simulink model "challenge1_2"  (R2022b)
settings: Solver=ode45  StartTime=0.0  StopTime=10  RelTol=1e-3
undefined symbols (not defined in the file or in its folder): awu, degs2rpm, der, end_step, pid, rpm2degs, sens, simul, Ts
libraries: simulink x4
settings Model: Creator=emanuelevitetta  LastModifiedBy=david

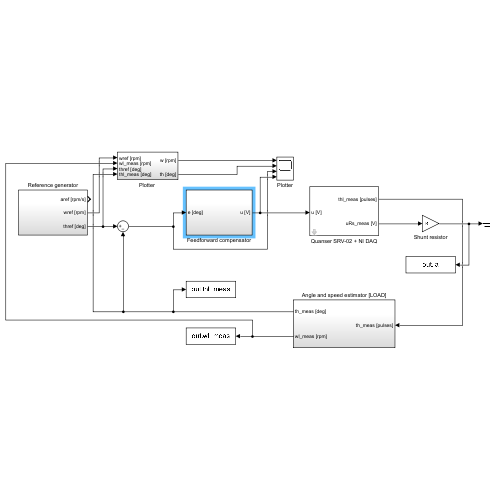
[thumbnail: Simulink's stored preview of the top-level diagram]
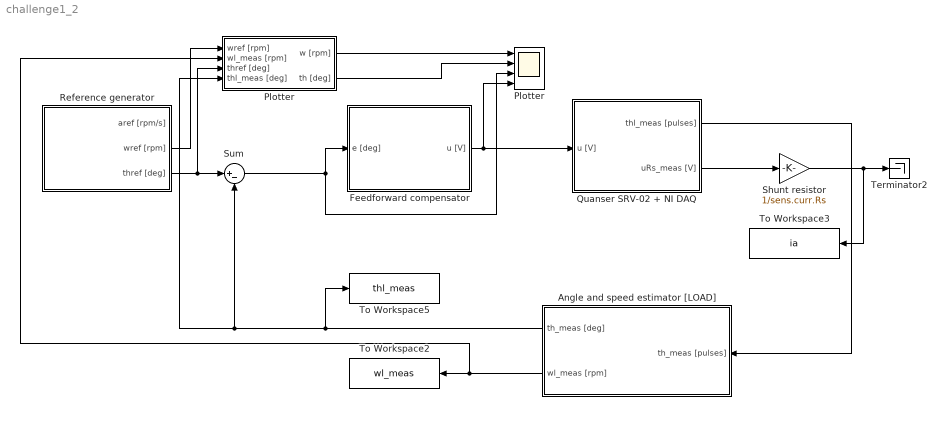
== system challenge1_2 ==
  Angle and speed estimator [LOAD] : Subsystem
  Feedforward compensator : Subsystem
  Plotter : Scope  NumInputPorts=4
  "Plotter " : Subsystem
  Quanser SRV-02 + NI DAQ : Subsystem  mask(Quanser SRV-02 (with inertial load) + NI DAQ){Ts=0.001, fricType=Coulomb + viscous}
      mask prompts: Ts "NI DAQ Sample Time:"; fricType "Friction model"
      mask help: Quanser SRV-02 (with inertial load) + NI DAQ model.
      mask init:
      | %%  Sensors data
      | 
      | %   shunt resistor
      | sens.curr.Rs = 0.5;                         %   resistance [Ohm]   
      | sens.curr.uRs_std = 0.01;                   %   voltage noise standard dev [V]                           
      | sens.curr.uRs_var = sens.curr.uRs_std^2;	%   voltage noise variance [V^2]
      | 
      | %   Hewlett-Packard HEDS-5540#A06 optical encoder
      | sens.enc.ppr = 500*4;                       %   pulses per rotation
      | sens.enc.pulse2deg = 360/sens.enc.ppr;      %   [pulses] -> [deg]
      | sens.enc.pulse2rad = 2*pi/sens.enc.ppr;     %   [pulses] -> [rad]
      | sens.enc.deg2pulse = sens.enc.ppr/360;      %   [deg] -> [pulses]
      | sens.enc.rad2pulse = sens.enc.ppr/2/pi;     %   [rad] -> [pulses]
      | 
      | 
      | %%  Data acquisition board (daq) data
      | 
      | %   NI PCI-6221 DAC data
      | daq.dac.bits = 16;                                  %   resolution (bits)
      | daq.dac.fs   = 10;                                  %   full scale 
      | daq.dac.q    = 2*daq.dac.fs/(2^daq.dac.bits-1);     %	quantization
      | 
      | %   NI PCI-6221 ADC data
      | daq.adc.bits = 16;                                  %   resolution (bits)
      | daq.adc.fs   = 10;                                  %   full scale (as set in SLDRT Analog Input block)
      | daq.adc.q    = 2*daq.adc.fs/(2^daq.adc.bits-1);     %   quantization
      mask Help:
      | Riccardo Antonello (antonello@dei.unipd.it)
      | 
      | April 24, 2020
      | 
      | Dept. of Information Engineering, University of Padova
      mask TypeOptions fricType: Coulomb + viscous | Karnopp
  Reference generator : Subsystem
  Shunt resistor : Gain  Gain=1/sens.curr.Rs
  Sum : Sum  Inputs=|+-
  Terminator2 : Terminator
  To Workspace2 : ToWorkspace  VariableName=wl_meas  SaveFormat=Structure With Time  SampleTime=Ts
  To Workspace3 : ToWorkspace  VariableName=ia  SaveFormat=Structure With Time  SampleTime=Ts
  To Workspace5 : ToWorkspace  VariableName=thl_meas  SaveFormat=Structure With Time  SampleTime=Ts
  wires:
  Quanser SRV-02 + NI DAQ/2(uRs_meas [V]) -> Shunt resistor/1
  Shunt resistor/1 -> To Workspace3/1, Terminator2/1
  Reference generator/3(thref [deg]) -> "Plotter "/3(thref [deg]), Sum/1
  Quanser SRV-02 + NI DAQ/1(thl_meas [pulses]) -> Angle and speed estimator [LOAD]/1(th_meas [pulses])
  Angle and speed estimator [LOAD]/1(th_meas [deg]) -> "Plotter "/4(thl_meas [deg]), Sum/2, To Workspace5/1
  Angle and speed estimator [LOAD]/2(wl_meas [rpm]) -> "Plotter "/2(wl_meas [rpm]), To Workspace2/1
  Reference generator/2(wref [rpm]) -> "Plotter "/1(wref [rpm])
  "Plotter "/1(w [rpm]) -> Plotter/1
  Feedforward compensator/1(u [V]) -> Quanser SRV-02 + NI DAQ/1(u [V]), Plotter/4
  Sum/1 -> Plotter/3, Feedforward compensator/1(e [deg])
  "Plotter "/2(th [deg]) -> Plotter/2

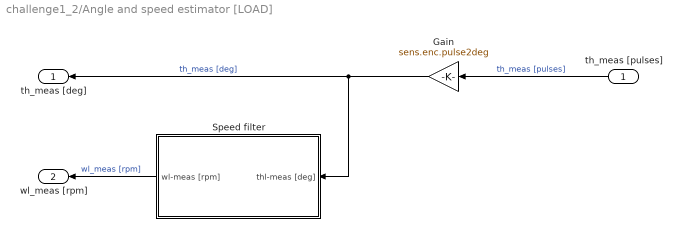
== system challenge1_2/Angle and speed estimator [LOAD] ==
  th_meas [pulses] : Inport
  Gain : Gain  Gain=sens.enc.pulse2deg
  Speed filter : Subsystem
  th_meas [deg] : Outport
  wl_meas [rpm] : Outport  Port=2
  wires:
  Speed filter/1(wl-meas [rpm]) -> wl_meas [rpm]/1  "wl_meas [rpm]"
  th_meas [pulses]/1 -> Gain/1  "th_meas [pulses]"
  Gain/1 -> Speed filter/1(thl-meas [deg]), th_meas [deg]/1  "th_meas [deg]"

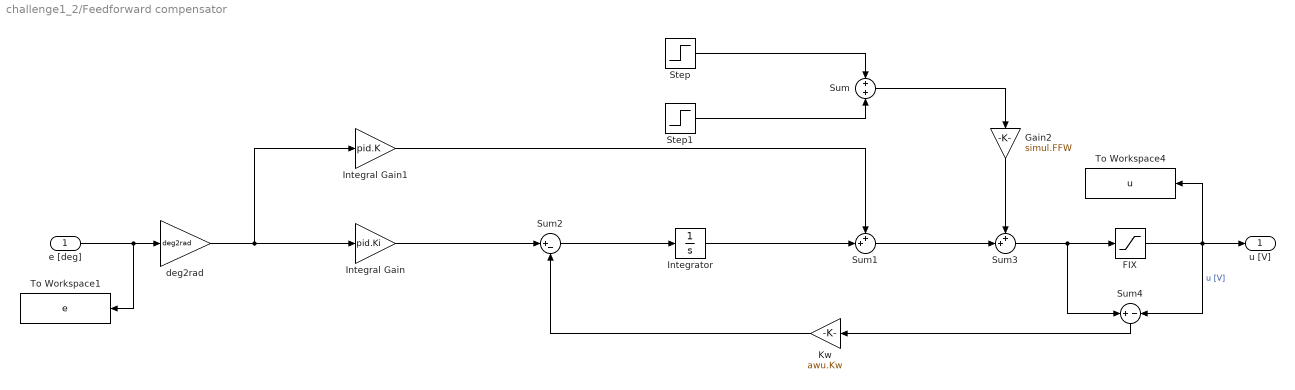
== system challenge1_2/Feedforward compensator ==
  e [deg] : Inport
  "FIX " : Saturate  UpperLimit=10  LowerLimit=-10
  Gain2 : Gain  Gain=simul.FFW
  Integral Gain : Gain  Gain=pid.Ki
  Integral Gain1 : Gain  Gain=pid.K
  Integrator : Integrator
  Kw : Gain  Gain=awu.Kw
  Step : Step  After=10  SampleTime=Ts
  Step1 : Step  Time=end_step  After=-10  SampleTime=Ts
  Sum : Sum
  Sum1 : Sum  Inputs=++|
  Sum2 : Sum  Inputs=|+-
  Sum3 : Sum  Inputs=++|
  Sum4 : Sum  Inputs=+-
  To Workspace1 : ToWorkspace  VariableName=e  SaveFormat=Structure With Time  SampleTime=Ts
  To Workspace4 : ToWorkspace  VariableName=u  SaveFormat=Structure With Time  SampleTime=Ts
  deg2rad : Gain  Gain=deg2rad
  u [V] : Outport
  wires:
  deg2rad/1 -> Integral Gain1/1, Integral Gain/1
  e [deg]/1 -> To Workspace1/1, deg2rad/1
  Gain2/1 -> Sum3/1
  Integrator/1 -> Sum1/2
  Step/1 -> Sum/1
  Step1/1 -> Sum/2
  Sum/1 -> Gain2/1
  Sum1/1 -> Sum3/2
  Integral Gain1/1 -> Sum1/1
  Sum3/1 -> Sum4/1, "FIX "/1
  "FIX "/1 -> Sum4/2, To Workspace4/1, u [V]/1  "u [V]"
  Integral Gain/1 -> Sum2/1
  Kw/1 -> Sum2/2
  Sum4/1 -> Kw/1
  Sum2/1 -> Integrator/1

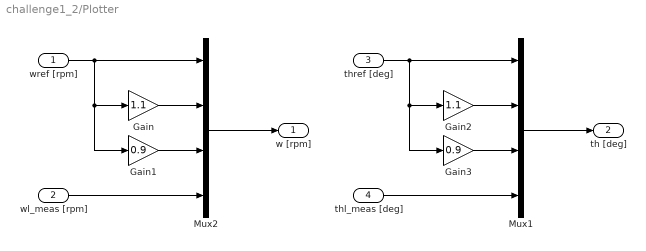
== system challenge1_2/Plotter  ==
  wref [rpm] : Inport
  wl_meas [rpm] : Inport  Port=2
  thref [deg] : Inport  Port=3
  thl_meas [deg] : Inport  Port=4
  Gain : Gain  Gain=1.1
  Gain1 : Gain  Gain=0.9
  Gain2 : Gain  Gain=1.1
  Gain3 : Gain  Gain=0.9
  Mux1 : Mux
  Mux2 : Mux
  w [rpm] : Outport
  th [deg] : Outport  Port=2
  wires:
  wref [rpm]/1 -> Gain1/1, Gain/1, Mux2/1
  Mux2/1 -> w [rpm]/1
  wl_meas [rpm]/1 -> Mux2/4
  Gain/1 -> Mux2/2
  Gain1/1 -> Mux2/3
  thref [deg]/1 -> Gain3/1, Gain2/1, Mux1/1
  thl_meas [deg]/1 -> Mux1/4
  Gain2/1 -> Mux1/2
  Gain3/1 -> Mux1/3
  Mux1/1 -> th [deg]/1

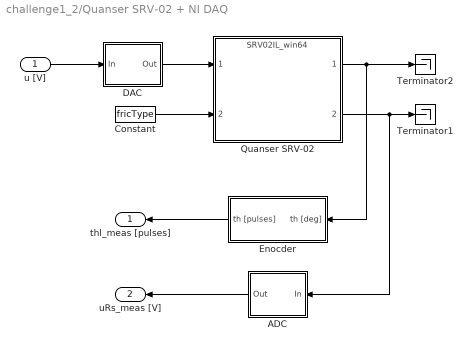
== system challenge1_2/Quanser SRV-02 + NI DAQ ==
  u [V] : Inport
  ADC : Subsystem
  Constant : Constant  Value=fricType
  DAC : Subsystem
  Enocder : Subsystem
  Quanser SRV-02 : ModelReference  ModelNameDialog=SRV02IL_win64.slxp  ModelReferenceVersion=1.44  CopyOfModelProtected=on
  Terminator1 : Terminator
  Terminator2 : Terminator
  thl_meas [pulses] : Outport
  uRs_meas [V] : Outport  Port=2
  wires:
  Enocder/1(th [pulses]) -> thl_meas [pulses]/1
  ADC/1(Out) -> uRs_meas [V]/1
  DAC/1(Out) -> Quanser SRV-02/1
  Quanser SRV-02/2 -> ADC/1(In), Terminator1/1
  u [V]/1 -> DAC/1(In)
  Quanser SRV-02/1 -> Enocder/1(th [deg]), Terminator2/1
  Constant/1 -> Quanser SRV-02/2

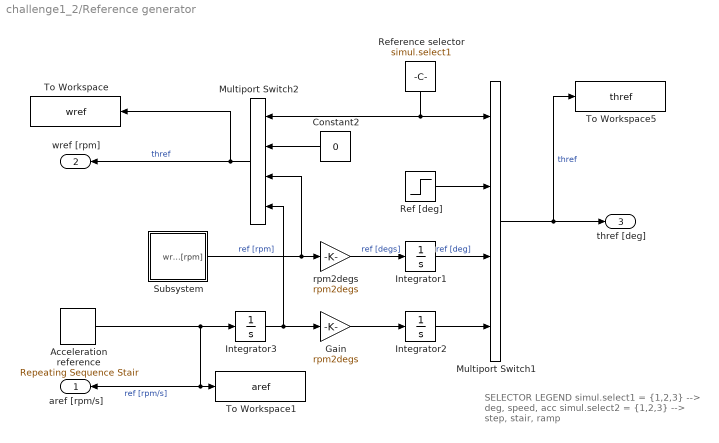
== system challenge1_2/Reference generator ==
  note: SELECTOR LEGEND
      |
      | simul.select1 = {1,2,3} --> deg, speed, acc
      | simul.select2 = {1,2,3} --> step, stair, ramp
  Acceleration reference : simulink/Sources/Repeating Sequence Stair  OutValues=[900 0 -900 -900 0 900].'  tsamp=0.5  OutMin=[]  OutMax=[]  OutDataTypeStr=double  OutputDataTypeScalingMode=double  OutDataType=fixdt(0,8)  ConRadixGroup=Best Precision: Vector-wise  OutScaling=2^-12
  Constant2 : Constant  Value=0
  Gain : Gain  Gain=rpm2degs
  Integrator1 : Integrator
  Integrator2 : Integrator
  Integrator3 : Integrator
  Multiport Switch1 : MultiPortSwitch  SaturateOnIntegerOverflow=off  InputSameDT=off
  Multiport Switch2 : MultiPortSwitch  SaturateOnIntegerOverflow=off  InputSameDT=off
  Ref [deg] : Step  After=simul.stepdeg
  Reference selector : Constant  Value=simul.select1
  Subsystem : Subsystem
  To Workspace : ToWorkspace  VariableName=wref  SaveFormat=Structure With Time  SampleTime=Ts
  To Workspace1 : ToWorkspace  VariableName=aref  SaveFormat=Structure With Time  SampleTime=Ts
  To Workspace5 : ToWorkspace  VariableName=thref  SaveFormat=Structure With Time  SampleTime=Ts
  rpm2degs : Gain  Gain=rpm2degs
  aref [rpm/s] : Outport
  wref [rpm] : Outport  Port=2
  thref [deg] : Outport  Port=3
  wires:
  Integrator1/1 -> Multiport Switch1/3  "ref [deg]"
  rpm2degs/1 -> Integrator1/1  "ref [degs]"
  Ref [deg]/1 -> Multiport Switch1/2
  Reference selector/1 -> Multiport Switch2/1, Multiport Switch1/1
  Multiport Switch1/1 -> To Workspace5/1, thref [deg]/1  "thref"
  Subsystem/1(wref [rpm]) -> Multiport Switch2/3, rpm2degs/1  "ref [rpm]"
  Integrator2/1 -> Multiport Switch1/4
  Gain/1 -> Integrator2/1
  Integrator3/1 -> Multiport Switch2/4, Gain/1
  Acceleration reference/1 -> Integrator3/1, aref [rpm/s]/1, To Workspace1/1  "ref [rpm/s]"
  Constant2/1 -> Multiport Switch2/2
  Multiport Switch2/1 -> wref [rpm]/1, To Workspace/1  "thref"

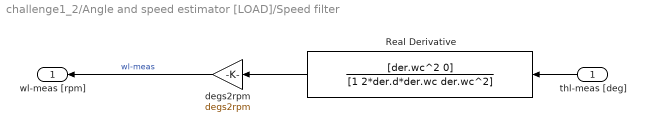
== system challenge1_2/Angle and speed estimator [LOAD]/Speed filter ==
  thl-meas [deg] : Inport
  Real Derivative : TransferFcn  Numerator=[der.wc^2 0]  Denominator=[1 2*der.d*der.wc der.wc^2]
  degs2rpm : Gain  Gain=degs2rpm
  wl-meas [rpm] : Outport
  wires:
  thl-meas [deg]/1 -> Real Derivative/1
  degs2rpm/1 -> wl-meas [rpm]/1  "wl-meas"
  Real Derivative/1 -> degs2rpm/1

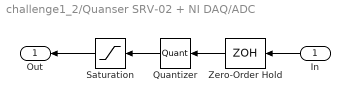
== system challenge1_2/Quanser SRV-02 + NI DAQ/ADC ==
  In : Inport
  Quantizer : Quantizer  QuantizationInterval=daq.adc.q
  Saturation : Saturate  UpperLimit=daq.adc.fs  LowerLimit=-daq.adc.fs
  Zero-Order Hold : ZeroOrderHold  SampleTime=Ts
  Out : Outport
  wires:
  Saturation/1 -> Out/1
  In/1 -> Zero-Order Hold/1
  Quantizer/1 -> Saturation/1
  Zero-Order Hold/1 -> Quantizer/1

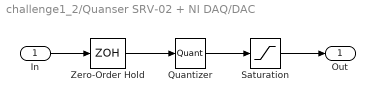
== system challenge1_2/Quanser SRV-02 + NI DAQ/DAC ==
  In : Inport
  Quantizer : Quantizer  QuantizationInterval=daq.dac.q
  Saturation : Saturate  UpperLimit=daq.dac.fs  LowerLimit=-daq.dac.fs
  Zero-Order Hold : ZeroOrderHold  SampleTime=Ts
  Out : Outport
  wires:
  Quantizer/1 -> Saturation/1
  In/1 -> Zero-Order Hold/1
  Zero-Order Hold/1 -> Quantizer/1
  Saturation/1 -> Out/1

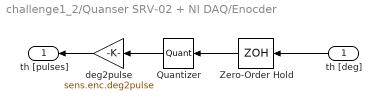
== system challenge1_2/Quanser SRV-02 + NI DAQ/Enocder ==
  th [deg] : Inport
  Quantizer : Quantizer  QuantizationInterval=sens.enc.pulse2deg
  Zero-Order Hold : ZeroOrderHold  SampleTime=Ts
  deg2pulse : Gain  Gain=sens.enc.deg2pulse
  th [pulses] : Outport
  wires:
  Quantizer/1 -> deg2pulse/1
  th [deg]/1 -> Zero-Order Hold/1
  Zero-Order Hold/1 -> Quantizer/1
  deg2pulse/1 -> th [pulses]/1

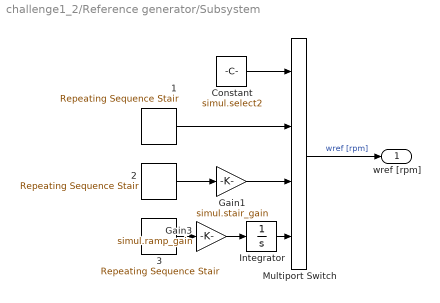
== system challenge1_2/Reference generator/Subsystem ==
  1 : simulink/Sources/Repeating Sequence Stair  OutValues=[250 -250].'  tsamp=1  OutMin=[]  OutMax=[]  OutDataTypeStr=double  OutputDataTypeScalingMode=double  OutDataType=fixdt(0,8)  ConRadixGroup=Best Precision: Vector-wise  OutScaling=2^-12
  2 : simulink/Sources/Repeating Sequence Stair  OutValues=[50 100 150 200 250 300 350 400 450 450].'  tsamp=5  OutMin=[]  OutMax=[]  OutDataTypeStr=double  OutputDataTypeScalingMode=double  OutDataType=fixdt(0,8)  ConRadixGroup=Best Precision: Vector-wise  OutScaling=2^-12
  3 : simulink/Sources/Repeating Sequence Stair  OutValues=[450 -450].'  tsamp=1  OutMin=[]  OutMax=[]  OutDataTypeStr=double  OutputDataTypeScalingMode=double  OutDataType=fixdt(0,8)  ConRadixGroup=Best Precision: Vector-wise  OutScaling=2^-12
  Constant : Constant  Value=simul.select2
  Gain1 : Gain  Gain=simul.stair_gain
  Gain3 : Gain  Gain=simul.ramp_gain
  Integrator : Integrator
  Multiport Switch : MultiPortSwitch  SaturateOnIntegerOverflow=off  InputSameDT=off
  wref [rpm] : Outport
  wires:
  1/1 -> Multiport Switch/2
  Gain3/1 -> Integrator/1
  Integrator/1 -> Multiport Switch/4
  Multiport Switch/1 -> wref [rpm]/1  "wref [rpm]"
  Gain1/1 -> Multiport Switch/3
  Constant/1 -> Multiport Switch/1
  3/1 -> Gain3/1
  2/1 -> Gain1/1
